simulink model "PassivityBasedControl"  (R2021a)
settings: Solver=FixedStepAuto  StartTime=0  StopTime=5  FixedStep=0.001  RelTol=1e-3
settings Model: Creator=negin  LastModifiedBy=negin

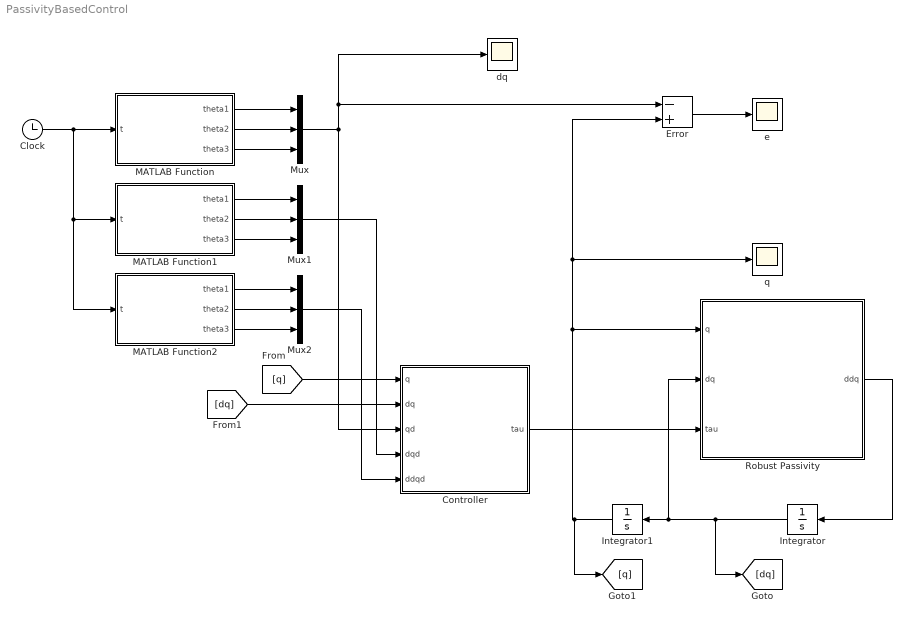
== system PassivityBasedControl ==
  Clock : Clock
      settings: Decimation=5
  Controller : MATLAB Function  TreatAsAtomicUnit=on
  Error : Sum  Inputs=-+
  Integrator : Integrator  InitialCondition=[0; 0; 0]
  Integrator1 : Integrator  InitialCondition=[0; 0; 0]
  MATLAB Function : MATLAB Function  TreatAsAtomicUnit=on
  MATLAB Function1 : MATLAB Function  TreatAsAtomicUnit=on
  MATLAB Function2 : MATLAB Function  TreatAsAtomicUnit=on
  Mux : Mux  Inputs=3
  Mux1 : Mux  Inputs=3
  Mux2 : Mux  Inputs=3
  Robust Passivity : MATLAB Function  TreatAsAtomicUnit=on
  dq : Scope
  e : Scope
  q : Scope
  wires:
  Robust Passivity/1(ddq) -> Integrator/1
  Integrator/1 -> [dq], Robust Passivity/2(dq), Integrator1/1
  Integrator1/1 -> [q], Robust Passivity/1(q), q/1, Error/2
  MATLAB Function/1(theta1) -> Mux/1
  Clock/1 -> MATLAB Function2/1(t), MATLAB Function1/1(t), MATLAB Function/1(t)
  MATLAB Function/2(theta2) -> Mux/2
  MATLAB Function/3(theta3) -> Mux/3
  Mux/1 -> dq/1, Error/1, Controller/3(qd)
  MATLAB Function1/1(theta1) -> Mux1/1
  MATLAB Function1/2(theta2) -> Mux1/2
  MATLAB Function1/3(theta3) -> Mux1/3
  MATLAB Function2/1(theta1) -> Mux2/1
  MATLAB Function2/2(theta2) -> Mux2/2
  MATLAB Function2/3(theta3) -> Mux2/3
  Error/1 -> e/1
  Controller/1(tau) -> Robust Passivity/3(tau)
  Mux2/1 -> Controller/5(ddqd)
  Mux1/1 -> Controller/4(dqd)
  [q] -> Controller/1(q)
  [dq] -> Controller/2(dq)

== matlab function PassivityBasedControl/MATLAB Function ==
  data: theta1 output; t input; theta2 output; theta3 output
function [theta1, theta2, theta3] = desiredTraj(t)
theta1 = 0.1309*t^2 + 0.0147*t^3 - 0.0085*t^4 + 0.0007*t^5;
theta2 = 0.1309*t^2 - 0.0188*t^3 - 0.001*t^4 + 0.0002*t^5;
theta3 = 0.1309*t^2 + 0.0314*t^3 - 0.0123*t^4 + 0.001*t^5;

== matlab function PassivityBasedControl/Robust Passivity ==
  data: q input; ddq output; dq input; tau input
function ddq = RobotDynamics(q, dq, tau)

m1 = 1;
m2 = 1;
m3 = 1;

l1 = 1;
l2 = 1;
l3 = 1;

r1 = l1/2;
r2 = l2/2;
r3 = l3/2;

R1 = 0.05;
R2 = 0.05;
R3 = 0.05;

g = 9.81;

a1 = m2*r2^2 + m3*l2^2;
a2 = m3*r3^2;
a3 = m3*r3*l2;
b1 = (m2*r2 + m3*l2)*g;
b2 = m3*r3*g;
I1 = 0.5*m1*R1^2;
I2 = 0.5*m2*R2^2;
I3 = 0.5*m3*R3^2;

M11 = a1*cos(q(2))^2 + a2*cos(q(2) + q(3))^2 + 2*a3*cos(q(2))*cos(q(2) + q(3)) + I1;
M12 = 0; 
M13 = 0; 
M21 = 0; 
M31 = 0;
M22 = a1 + a2 + 2*a3*cos(q(3)) + I2;
M23 = a2 + a3*cos(q(3));
M32 = a2 + a3*cos(q(3));
M33 = a2 + I3;
M = [M11 M12 M13; M21 M22 M23; M31 M32 M33];

C11 = -0.5*a1*dq(2)*sin(2*q(2)) - 0.5*a2*(dq(2) + dq(3))*sin(2*q(2) + 2*q(3))...
    - a3*dq(2)*sin(2*q(2) + q(3)) - a3*dq(3)*cos(q(2))*sin(q(2) + q(3));
C12 = -0.5*a1*dq(1)*sin(2*q(2)) - 0.5*a2*dq(1)*sin(2*q(2) + 2*q(3)) - ...
    a3*dq(1)*sin(2*q(2) + q(3));
C13 = -0.5*a2*dq(1)*sin(2*q(2) + 2*q(3)) - a3*dq(1)*cos(q(2))*sin(q(2) + q(3));
C21 = -C12;
C22 = -a3*dq(3)*sin(q(3));
C23 = -a3*(dq(2) + dq(3))*sin(q(3));
C31 = -C13;
C32 = a3*dq(2)*sin(q(3));
C33 = 0;
C = [C11 C12 C13; C21 C22 C23; C31 C32 C33];

G11 = 0;
G21 = m2*l2*sin(q(2))*g/2 - m3*l3*sin(q(2) + q(3))*g/2 - m3*l2*sin(q(2))*g;
G31 = -m3*l3*sin(q(2) + q(3))*g/2;
G = [G11; G21; G31];

ddq = inv(M)*(tau - C*dq - G);
end

== matlab function PassivityBasedControl/Controller ==
  data: q input; tau output; dq input; qd input; dqd input; ddqd input
function tau = Controller(q, dq, qd, dqd, ddqd)

m1 = 1;
m2 = 1;
m3 = 1;

l1 = 1;
l2 = 1;
l3 = 1;

r1 = l1/2;
r2 = l2/2;
r3 = l3/2;

R1 = 0.05;
R2 = 0.05;
R3 = 0.05;

g = 9.81;

a1 = m2*r2^2 + m3*l2^2;
a2 = m3*r3^2;
a3 = m3*r3*l2;
b1 = (m2*r2 + m3*l2)*g;
b2 = m3*r3*g;
I1 = 0.5*m1*R1^2;
I2 = 0.5*m2*R2^2;
I3 = 0.5*m3*R3^2;

M11 = a1*cos(q(2))^2 + a2*cos(q(2) + q(3))^2 + 2*a3*cos(q(2))*cos(q(2) + q(3)) + I1;
M12 = 0; 
M13 = 0; 
M21 = 0; 
M31 = 0;
M22 = a1 + a2 + 2*a3*cos(q(3)) + I2;
M23 = a2 + a3*cos(q(3));
M32 = a2 + a3*cos(q(3));
M33 = a2 + I3;
M = [M11 M12 M13; M21 M22 M23; M31 M32 M33];

C11 = -0.5*a1*dq(2)*sin(2*q(2)) - 0.5*a2*(dq(2) + dq(3))*sin(2*q(2) + 2*q(3))...
    - a3*dq(2)*sin(2*q(2) + q(3)) - a3*dq(3)*cos(q(2))*sin(q(2) + q(3));
C12 = -0.5*a1*dq(1)*sin(2*q(2)) - 0.5*a2*dq(1)*sin(2*q(2) + 2*q(3)) - ...
    a3*dq(1)*sin(2*q(2) + q(3));
C13 = -0.5*a2*dq(1)*sin(2*q(2) + 2*q(3)) - a3*dq(1)*cos(q(2))*sin(q(2) + q(3));
C21 = -C12;
C22 = -a3*dq(3)*sin(q(3));
C23 = -a3*(dq(2) + dq(3))*sin(q(3));
C31 = -C13;
C32 = a3*dq(2)*sin(q(3));
C33 = 0;
C = [C11 C12 C13; C21 C22 C23; C31 C32 C33];

G11 = 0;
G21 = m2*l2*sin(q(2))*g/2 - m3*l3*sin(q(2) + q(3))*g/2 - m3*l2*sin(q(2))*g;
G31 = -m3*l3*sin(q(2) + q(3))*g/2;
G = [G11; G21; G31];

gamma = 0.1.*[1 0 0; 0 1 0; 0 0 1];
K = 0.01.*[1 1 1; 0 1 0; 0 0 1];

tau = M*(ddqd - gamma*(dq - dqd)) + C*(dqd - gamma*(q - qd)) + G + K*(dq - dqd + gamma*(q - qd));

end

== matlab function PassivityBasedControl/MATLAB Function1 ==
  data: theta1 output; t input; theta2 output; theta3 output
function [theta1, theta2, theta3] = ddesiredTraj(t)
theta1 = 0.1309*2*t + 0.0147*3*t^2 - 0.0085*4*t^3 + 0.0007*5*t^4;
theta2 = 0.1309*2*t - 0.0188*3*t^2 - 0.001*4*t^3 + 0.0002*5*t^4;
theta3 = 0.1309*2*t + 0.0314*3*t^2 - 0.0123*4*t^3 + 0.001*5*t^4;

== matlab function PassivityBasedControl/MATLAB Function2 ==
  data: theta1 output; t input; theta2 output; theta3 output
function [theta1, theta2, theta3] = dddesiredTraj(t)
theta1 = 0.1309*2 + 0.0147*3*2*t - 0.0085*4*3*t^2 + 0.0007*5*4*t^3;
theta2 = 0.1309*2 - 0.0188*3*2*t - 0.001*4*3*t^2 + 0.0002*5*4*t^3;
theta3 = 0.1309*2 + 0.0314*3*2*t - 0.0123*4*3*t^2 + 0.001*5*4*t^3;
